simulink model "Simulink_P7"  (R2025b)
settings: Solver=VariableStepAuto  StartTime=0.0  StopTime=2  RelTol=1e-3
InitFcn:
  | Ra = 2;
  | Kt = 0.01;
  | b = 0.0012;
  | La = 0.023;
  | Ke = 0.01;
  | J = 0.001;
  | Va = 24;

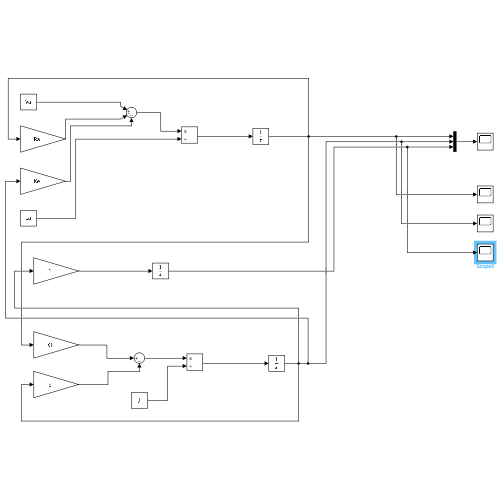
[thumbnail: Simulink's stored preview of the top-level diagram]
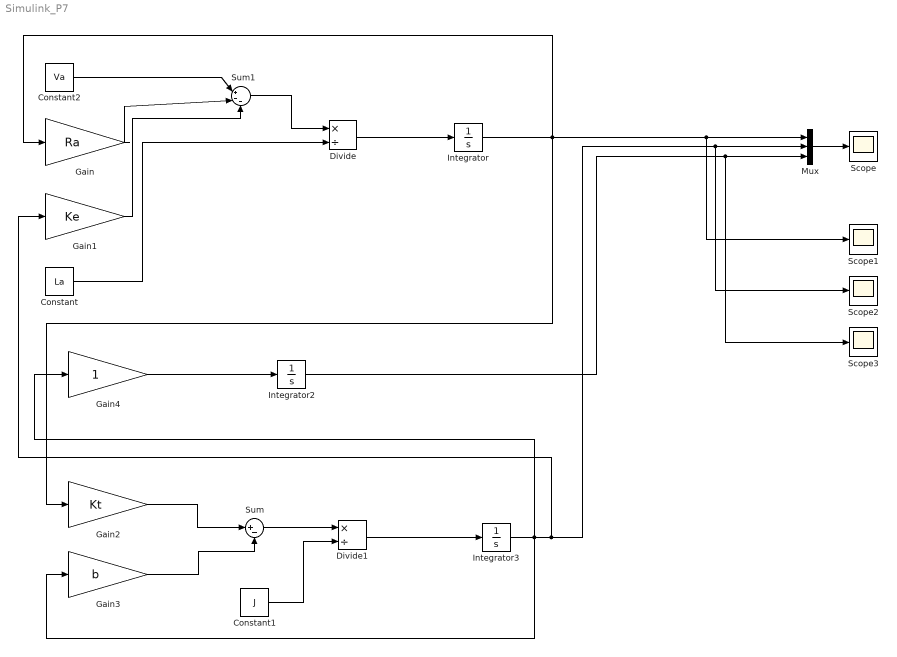
== system Simulink_P7 ==
  Constant : Constant  Value=La
  Constant1 : Constant  Value=J
  Constant2 : Constant  Value=Va
  Divide : Product  Inputs=*/
  Divide1 : Product  Inputs=*/
  Gain : Gain  Gain=Ra
  Gain1 : Gain  Gain=Ke
  Gain2 : Gain  Gain=Kt
  Gain3 : Gain  Gain=b
  Gain4 : Gain
  Integrator : Integrator
  Integrator2 : Integrator
  Integrator3 : Integrator
  Mux : Mux  Inputs=3
  Scope{,1..3} (4 alike) : Scope
      Scope settings: ActiveDisplayYMinimum=-59.58516129983083  ActiveDisplayYMaximum=124.6004233910671
      Scope1 settings: ActiveDisplayYMinimum=-59.58516129983083  ActiveDisplayYMaximum=124.6004233910671
      Scope2 settings: ActiveDisplayYMinimum=-59.58516129983083  ActiveDisplayYMaximum=124.6004233910671  DataLoggingVariableName=ScopeData2
      Scope3 settings: ActiveDisplayYMinimum=-59.58516129983083  ActiveDisplayYMaximum=124.6004233910671  DataLoggingVariableName=ScopeData3
  Sum : Sum  Inputs=|+-
  Sum1 : Sum  Inputs=|+--
  wires:
  Divide/1 -> Integrator/1
  Mux/1 -> Scope/1
  Integrator/1 -> Gain2/1, Gain/1, Scope1/1, Mux/1
  Constant/1 -> Divide/2
  Sum1/1 -> Divide/1
  Constant2/1 -> Sum1/1
  Gain/1 -> Sum1/2
  Gain1/1 -> Sum1/3
  Divide1/1 -> Integrator3/1
  Integrator3/1 -> Gain4/1, Gain3/1, Gain1/1, Scope2/1, Mux/2
  Sum/1 -> Divide1/1
  Constant1/1 -> Divide1/2
  Gain3/1 -> Sum/2
  Gain2/1 -> Sum/1
  Gain4/1 -> Integrator2/1
  Integrator2/1 -> Scope3/1, Mux/3
